simulink model "atmoDrag_test"  (R2018b)
settings: Solver=VariableStepAuto  StartTime=0.0  StopTime=10.0  RelTol=1e-3
undefined symbols (not defined in the file or in its folder): u_h, vrel
libraries: atmoDrag_lib x1, time_Lib x1
settings Model: Creator=devantormey  LastModifiedBy=Kate

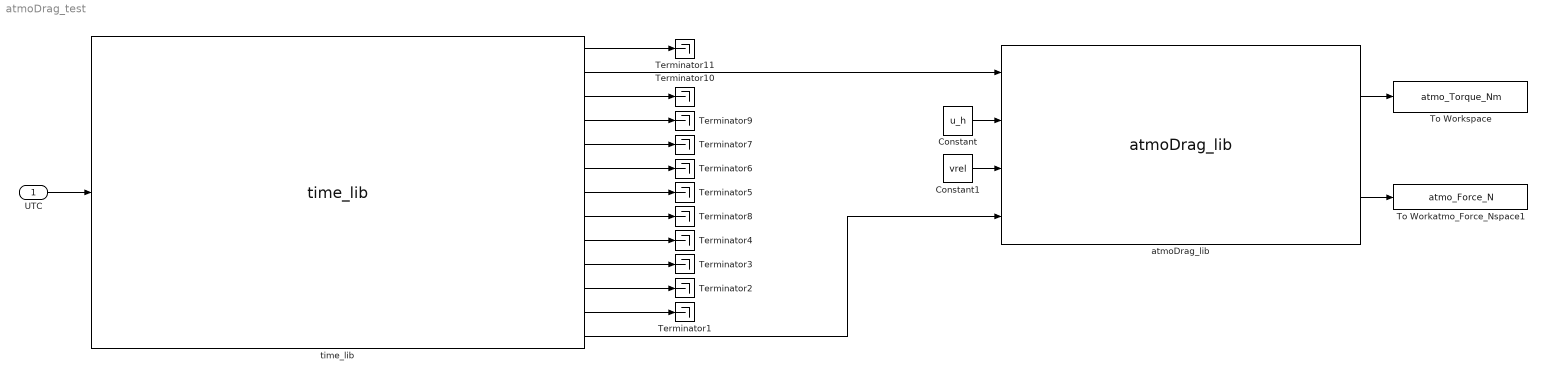
== system atmoDrag_test ==
  UTC : Inport
  Constant : Constant  Value=u_h
  Constant1 : Constant  Value=vrel
  Terminator{1..11} (11 alike) : Terminator
  To Workatmo_Force_Nspace1 : ToWorkspace  VariableName=atmo_Force_N  SaveFormat=Timeseries  SampleTime=-1
  To Workspace : ToWorkspace  VariableName=atmo_Torque_Nm  SaveFormat=Timeseries  SampleTime=-1
  atmoDrag_lib : atmoDrag_lib/atmoDrag_lib  SystemSampleTime=-1
  "time_lib " : time_Lib/time_lib    SystemSampleTime=-1
  wires:
  "time_lib "/7 -> Terminator5/1
  UTC/1 -> "time_lib "/1
  "time_lib "/10 -> Terminator3/1
  "time_lib "/12 -> Terminator1/1
  "time_lib "/11 -> Terminator2/1
  "time_lib "/8 -> Terminator8/1
  "time_lib "/3 -> Terminator10/1
  "time_lib "/5 -> Terminator7/1
  "time_lib "/4 -> Terminator9/1
  "time_lib "/1 -> Terminator11/1
  "time_lib "/6 -> Terminator6/1
  "time_lib "/9 -> Terminator4/1
  "time_lib "/2 -> atmoDrag_lib/1
  "time_lib "/13 -> atmoDrag_lib/4
  Constant/1 -> atmoDrag_lib/2
  Constant1/1 -> atmoDrag_lib/3
  atmoDrag_lib/1 -> To Workspace/1
  atmoDrag_lib/2 -> To Workatmo_Force_Nspace1/1
